simulink model "base_model_lqeH"  (R2020b)
settings: Solver=ode1  StartTime=0  StopTime=1150  FixedStep=0.1  RelTol=1e-3
libraries: simulink_extras x33
(part 3 of 3)

== matlab function base_model_lqeH/seter11 ==
  data: signal output size=1; time_shift input
function signal  = slowData(time_shift)
  
    persistent time_mem

    if isempty(time_mem)
        time_mem = 0;
    end
    
    signal = 0;
    time_mem = time_mem + time_shift;
    
    if time_mem >= 1
        signal = 1;
        time_mem = 0;
    end
    
end

== matlab function base_model_lqeH/seter12 ==
  data: signal output size=1; time_shift input
function signal  = slowData(time_shift)
  
    persistent time_mem

    if isempty(time_mem)
        time_mem = 0;
    end
    
    signal = 0;
    time_mem = time_mem + time_shift;
    
    if time_mem >= 1
        signal = 1;
        time_mem = 0;
    end
    
end

== matlab function base_model_lqeH/seter13 ==
  data: signal output size=1; time_shift input
function signal  = slowData(time_shift)
  
    persistent time_mem

    if isempty(time_mem)
        time_mem = 0;
    end
    
    signal = 0;
    time_mem = time_mem + time_shift;
    
    if time_mem >= 1
        signal = 1;
        time_mem = 0;
    end
    
end

== matlab function base_model_lqeH/MATLAB Function3 ==
  data: GRS output; ACC output; heading output; pitch output; roll output; lat output; lon output; Ve output; Vn output; H output; Vh output; time_shft output; cntrl_data output; lat_off output; lon_off output; alt_off output; Ve_off output; Vn_off output; Vh_off output; satStart output; satStop output; satDeltaUp output; satDeltaDown output
function [GRS, ACC, heading, pitch, roll, lat, lon, Ve, Vn,  H, Vh, time_shft,cntrl_data,...
          lat_off, lon_off, alt_off, Ve_off, Vn_off,  Vh_off,...
          satStart, satStop, satDeltaUp, satDeltaDown] = fcn


persistent i data time_mem dataOS cntrl_data_mem
%ini_model

if isempty(i)
    i = 5;
    data   = load('im_100hz_type_0_ref.mat');
%     data   = load('wave-3.0m-150s-250s.mat'); %'wave-1.0m-100s-200s.mat'
    dataOS = load('im_100hz_type_0_ref.mat');%'ramp-0.5ms-150s-300s.mat'
    
    time_mem = data.time(i) - (data.time(i+1) - data.time(i));
    
%    cntrl_data_mem = [data.Ve(i+1); data.Vn(i+1);data.Vh(i+1);...
%                      data.lat(i+1);data.lon(i+1);data.H(i+1);...   
%                      data.heading(i+1); data.pitch(i+1); data.roll(i+1)];
                      
end

GRS =  data.tied_grs(i,:)';%data.grs(i,:)';
ACC =  data.tied_acc(i,:)';%data.acc(i,:)';

heading = data.heading(i);
pitch   = data.pitch(i);
roll    = data.roll(i);

time_shft = data.time(i) - time_mem;
time_mem  = data.time(i);


Ve = data.lla_vel(i,2);
Vn = data.lla_vel(i,1);
Vh = data.lla_vel(i,3);

lat = data.lla_pos(i,1);
lon = data.lla_pos(i,2);
H   = data.lla_pos(i,3);





% Ve = data.Ve(i);
% Vn = data.Vn(i);
% Vh = data.Vh(i);
% 
% 
% lat = data.latitude(i);
% lon = data.longitude(i);
% H   = data.altitude(i);

% if time_mem < 145/  time_shft
%     Ve_off = data.lla_vel(i,2);
%     Vn_off = data.lla_vel(i,1);
%     Vh_off = data.lla_vel(i,3);
% 
%     lat_off = data.lla_pos(i,1);
%     lon_off = data.lla_pos(i,2);
%     alt_off = data.lla_pos(i,3);
% else
    Ve_off = dataOS.lla_vel(i,2);
    Vn_off = dataOS.lla_vel(i,1);
    Vh_off = dataOS.lla_vel(i,3);

    lat_off = dataOS.lla_pos(i,1);
    lon_off = dataOS.lla_pos(i,2);
    alt_off = dataOS.lla_pos(i,3);
% end

cntrl_data = [data.lla_vel(i+1,2); data.lla_vel(i+1,1);data.lla_vel(i+1,3);...
                      data.lla_pos(i+1,1);data.lla_pos(i+1,2);data.lla_pos(i+1,3);...   
                      data.heading(i+1); data.pitch(i+1); data.roll(i+1)];

% cntrl_data = [data.Ve(i+1); data.Vn(i+1);data.Vh(i+1);...
%                       data.latitude(i+1);data.longitude(i+1);data.altitude(i+1);...   
%                       data.heading(i+1); data.pitch(i+1); data.roll(i+1)];

i = i + 1;  



% lat_off = dataOS.latitude(i);
% lon_off = dataOS.longitude(i);
% alt_off = dataOS.altitude(i);
% Ve_off  = dataOS.Ve(i);
% Vn_off  = dataOS.Vn(i);
% Vh_off  = dataOS.Vh(i);

satStart  = 0;
satStop   = 10000;
satDeltaUp = 0;
satDeltaDown = 0;

% if length(data.time)/100 < 1000
% %Traj type 1
%     satStart     = 30;
%     satDeltaUp   = 50;
% %     satStop      = 370;
% %     satDeltaDown = 200;
% else
%    %Traj type 2 
%     satStart     = 30;
%     satDeltaUp   = 300;
%     satStop      = 850;
%     satDeltaDown = 200;
% end
end

== matlab function base_model_lqeH/GNNS_freq_imitetor1 ==
  data: dispSatReal output; dispSat input; satStart input size=1; satStop input size=1; satDeltaUp input; satDeltaDown input; timeStep input
function dispSatReal = getDGSK(dispSat, satStart, satStop, satDeltaUp, satDeltaDown, timeStep)

    persistent timer
    if isempty(timer)
        timer = 0;
    end
    timer = timer + timeStep;
    dispSatReal = dispSat;
   
    if timer > satStart
        
        if timer < satStart + satDeltaUp
            dispSatReal = dispSat * 3;
        end
        if timer> satStop && timer < satStop + satDeltaDown
            dispSatReal = dispSat * 3;
        end
    end
    
    
    
end

== matlab function base_model_lqeH/Fuck matlab1 ==
  data: data_fix output; data input; criteria input; satCountPreset input
function data_fix =  forCtrl(data, criteria, satCountPreset)
    
    for ii = 1:1
        if data(ii) > criteria
            data(ii) = nan;
        end
    end
    data_fix = data;    
end

== matlab function base_model_lqeH/MATLAB Function4 ==
  data: GRS output; ACC output; heading output; pitch output; roll output; lat output; lon output; Ve output; Vn output; H output; Vh output; time_shft output; cntrl_data output; lat_off output; lon_off output; alt_off output; Ve_off output; Vn_off output; Vh_off output; satStart output; satStop output; satDeltaUp output; satDeltaDown output; corruptSatCount output; corruptTimeStart output; corruptPSDError output; corruptErrorType output; K_fastCircle_psd output; K_fastCircle_psd_dot output; K_slowWindow output; K_slowSensivity output
function [GRS, ACC, heading, pitch, roll, lat, lon, Ve, Vn,  H, Vh, time_shft,cntrl_data,...
          lat_off, lon_off, alt_off, Ve_off, Vn_off,  Vh_off,...
          satStart, satStop, satDeltaUp, satDeltaDown,...
          corruptSatCount, corruptTimeStart,corruptPSDError, corruptErrorType,...
          K_fastCircle_psd, K_fastCircle_psd_dot, K_slowWindow, K_slowSensivity]= fcn


persistent i data % time_mem dataOS cntrl_data_mem
%ini_model

if isempty(i)
    i = 5;
   data   = load('Z:\track_normal.mat');
%     data   = load('wave-3.0m-150s-250s.mat'); %'wave-1.0m-100s-200s.mat'
   % dataOS = load('im_100hz_type_0_ref.mat');%'ramp-0.5ms-150s-300s.mat'
    
%     time_mem = data.time(i) - (data.time(i+1) - data.time(i));
    
%    cntrl_data_mem = [data.Ve(i+1); data.Vn(i+1);data.Vh(i+1);...
%                      data.lat(i+1);data.lon(i+1);data.H(i+1);...   
%                      data.heading(i+1); data.pitch(i+1); data.roll(i+1)];
                      
end

GRS =  data.grs(: , i + 1);%data.tied_grs(i,:)';%data.grs(i,:)';
ACC =  data.acc(: , i + 1);%data.tied_acc(i,:)';%data.acc(i,:)';

heading = data.hdg(i);%data.heading(i);
pitch   = data.pth(i);%data.pitch(i);
roll    = data.rll(i);%data.roll(i);

time_shft = data.timeStep;%data.time(i) - time_mem;
% time_mem  = data.timeStamp;%data.time(i);


Ve = data.Ve(i);%data.lla_vel(i,2);
Vn = data.Vn(i);%data.lla_vel(i,1);
Vh = data.Vh(i);%data.lla_vel(i,3);

lat = data.lat(i);%data.lla_pos(i,1);
lon = data.lon(i);%data.lla_pos(i,2);
H   = data.alt(i);%data.lla_pos(i,3);

Ve_off = data.Ve(i);%data.lla_vel(i,2);
Vn_off = data.Vn(i);%data.lla_vel(i,1);
Vh_off = data.Vh(i);%data.lla_vel(i,3);

lat_off = data.lat(i);%data.lla_pos(i,1);
lon_off = data.lon(i);%data.lla_pos(i,2);
alt_off = data.alt(i);%data.lla_pos(i,3);

corruptSatCount  = data.corruptSatCount;
corruptTimeStart = data.corruptTimeStart;
corruptPSDError  = data.corruptPSDError;
corruptErrorType = data.corruptErrorType;

K_fastCircle_psd     = data.K_fastCircle_psd;
K_fastCircle_psd_dot = data.K_fastCircle_psd_dot;
K_slowWindow         = data.K_slowWindow;
K_slowSensivity      = data.K_slowSensivity;



cntrl_data = [ data.Ve(i+1);  data.Vn(i+1);  data.Vh(i+1);...
               data.lat(i+1); data.lon(i+1); data.alt(i+1);...   
               data.hdg(i+1); data.pth(i+1); data.rll(i+1)];

i = i + 1;           
           
% cntrl_data = [data.Ve(i+1); data.Vn(i+1);data.Vh(i+1);...
%                       data.latitude(i+1);data.longitude(i+1);data.altitude(i+1);...   
%                       data.heading(i+1); data.pitch(i+1); data.roll(i+1)];


% lat_off = dataOS.latitude(i);
% lon_off = dataOS.longitude(i);
% alt_off = dataOS.altitude(i);
% Ve_off  = dataOS.Ve(i);
% Vn_off  = dataOS.Vn(i);
% Vh_off  = dataOS.Vh(i);

satStart  = 0;
satStop   = data.timeDuration + data.timeDuration*0.1;
satDeltaUp = 0;
satDeltaDown = 0;



% if length(data.time)/100 < 1000
% %Traj type 1
%     satStart     = 30;
%     satDeltaUp   = 50;
% %     satStop      = 370;
% %     satDeltaDown = 200;
% else
%    %Traj type 2 
%     satStart     = 30;
%     satDeltaUp   = 300;
%     satStop      = 850;
%     satDeltaDown = 200;
% end
end

== matlab function base_model_lqeH/bigHeadingFix1 ==
  data: heading_bad input; heading_norm output
function heading_norm  = fix2PIerr (heading_bad)
    
    while (heading_bad < 0)
        heading_bad = heading_bad + 2*pi;
    end
    
    while (heading_bad > 2*pi)
        heading_bad = heading_bad - 2*pi;
    end
    
    
    heading_norm = heading_bad;
% 
% 
%     persistent headingError_mem
%     if isempty(headingError_mem)
%         headingError_mem = headingError;
%     end
%     fix_headingError = headingError;
%     if abs(fix_headingError) > 0.95*(2*3.1415)
%         fix_headingError = headingError_mem;
%     else
%         headingError_mem = headingError;    
%     end
end

== matlab function base_model_lqeH/Fuck matlab3 ==
  data: data_fix output size=8; data input; criteria input; satCountPreset input
function data_fix =  forCtrl(data, criteria, satCountPreset)
    
    data_fix = zeros(8,1);
    for ii = 1:8
        if data(ii) > criteria
            data(ii) = nan;
        end
    end
    data_fix = data;    
end

== matlab function base_model_lqeH/Fuck matlab4 ==
  data: data_fix output size=8; data input; criteria input; satCountPreset input
function data_fix =  forCtrl(data, criteria, satCountPreset)
    
    data_fix = zeros(8,1);
    for ii = 1:8
        if data(ii) > criteria
            data(ii) = nan;
        end
    end
    data_fix = data;    
end
